simulink library "Tube_Alpha"  (R2019b)
settings: Solver=ode45  StartTime=0.0  StopTime=10.0  RelTol=1e-3  EnableMultiTasking=on
undefined symbols (not defined in the file): Tube
libraries: simulink x1
settings Model: Creator=mbrauer  LastModifiedBy=bhisma
settings DataIOCC: LimitDataPoints=on  SaveFormat=Array  SignalLoggingSaveFormat=ModelDataLogs  ReturnWorkspaceOutputs=off
settings OptimizationCC: LifeSpan=inf
settings DebuggingCC: UnderspecifiedInitializationDetection=Classic  MergeDetectMultiDrivingBlocksExec=none  SolverPrmCheckMsg=warning  MultiTaskDSMMsg=warning  MultiTaskCondExecSysMsg=none  SFUnexpectedBacktrackingDiag=warning  SFNoUnconditionalDefaultTransitionDiag=warning  SFExecutionAtInitializationDiag=none  ArithmeticOperatorsInVariantConditions=warning
settings HardwareCC: ProdBitPerPointer=32  ProdBitPerSizeT=32  ProdBitPerPtrDiffT=32  ProdLargestAtomicFloat=None  ProdIntDivRoundTo=Undefined  ProdEndianess=Unspecified  ProdWordSize=32  ProdHWDeviceType=32-bit Generic
settings ModelReferenceCC: PropagateSignalLabelsOutOfModel=off
settings SFSimCC: SimUseLocalCustomCode=off  CustomCodeUndefinedFunction=UseInterfaceOnly
settings RTWCC: RTWUseLocalCustomCode=off
settings CodeAppCC: StateflowObjectComments=on
settings GRTTargetCC: TargetLangStandard=C89/C90 (ANSI)  GeneratePreprocessorConditionals=Disable all
settings ConfigComp: CovMetricSettings=dw  CovHtmlReporting=on  CovSaveCumulativeToWorkspaceVar=on  CovSaveSingleToWorkspaceVar=on  CovExternalEMLEnable=off

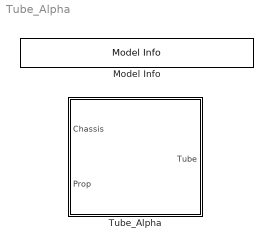
== system Tube_Alpha ==
  Model Info : simulink/Model-Wide Utilities/Model Info  Frame=on  DisplayStringWithTags=Copyright 2013-2014 The MathWorks, Inc.  HorizontalTextAlignment=Center  LeftAlignmentValue=0.5
  Tube_Alpha : Subsystem  VariantControl=VAR_Tube_Alpha

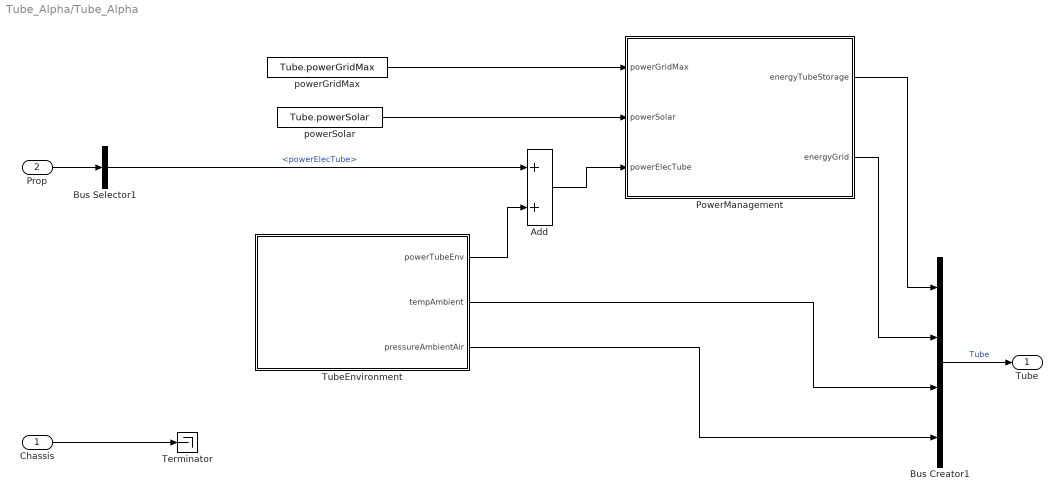
== system Tube_Alpha/Tube_Alpha ==
  Chassis : Inport
  Prop : Inport  Port=2
  Add : Sum
  Bus Creator1 : BusCreator  Inputs=4  NonVirtualBus=on
  Bus Selector1 : BusSelector  OutputSignals=powerElecTube
  PowerManagement : Subsystem
  Terminator : Terminator
  TubeEnvironment : Subsystem
  powerGridMax : Constant  Value=Tube.powerGridMax
  powerSolar : Constant  Value=Tube.powerSolar
  Tube : Outport
  wires:
  TubeEnvironment/2(tempAmbient) -> Bus Creator1/3
  Bus Creator1/1 -> Tube/1  "Tube"
  PowerManagement/1(energyTubeStorage) -> Bus Creator1/1
  Prop/1 -> Bus Selector1/1
  TubeEnvironment/1(powerTubeEnv) -> Add/2
  PowerManagement/2(energyGrid) -> Bus Creator1/2
  TubeEnvironment/3(pressureAmbientAir) -> Bus Creator1/4
  powerSolar/1 -> PowerManagement/2(powerSolar)
  powerGridMax/1 -> PowerManagement/1(powerGridMax)
  Bus Selector1/1 -> Add/1  "<powerElecTube>"
  Add/1 -> PowerManagement/3(powerElecTube)
  Chassis/1 -> Terminator/1

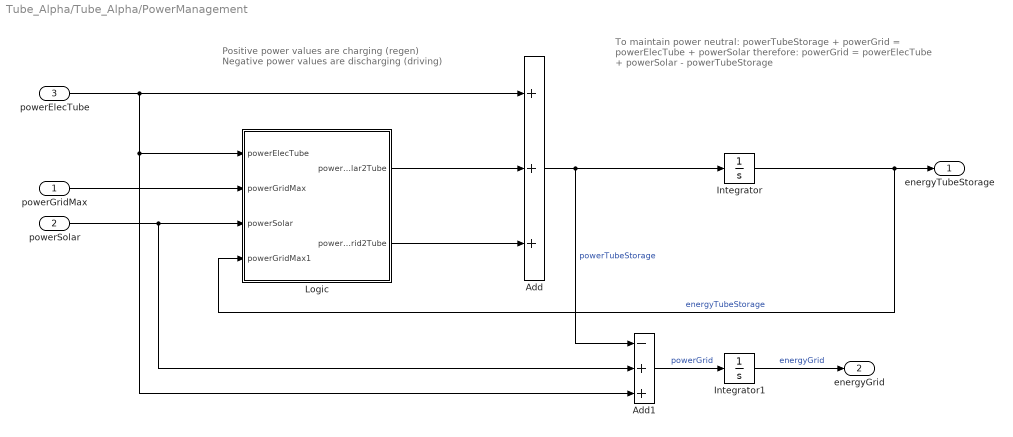
== system Tube_Alpha/Tube_Alpha/PowerManagement ==
  note: To maintain power neutral:
      | powerTubeStorage + powerGrid = powerElecTube + powerSolar
      |
      | therefore:
      | powerGrid = powerElecTube + powerSolar - powerTubeStorage
  note: Positive power values are charging (regen)
      | Negative power values are discharging (driving)
  powerGridMax : Inport
  powerSolar : Inport  Port=2
  powerElecTube : Inport  Port=3
  Add : Sum  Inputs=+++
  Add1 : Sum  Inputs=-++
  Integrator : Integrator  InitialCondition=Tube.energyStorage
      settings: AttributesFormatString=IC = %<InitialCondition>
  Integrator1 : Integrator
      settings: AttributesFormatString=IC = %<InitialCondition>
  Logic : Subsystem
  energyTubeStorage : Outport
  energyGrid : Outport  Port=2
  wires:
  Add/1 -> Integrator/1, Add1/1  "powerTubeStorage"
  Integrator1/1 -> energyGrid/1  "energyGrid"
  powerElecTube/1 -> Add1/3, Logic/1(powerElecTube), Add/1
  Integrator/1 -> Logic/4(powerGridMax1), energyTubeStorage/1  "energyTubeStorage"
  powerSolar/1 -> Add1/2, Logic/3(powerSolar)
  Add1/1 -> Integrator1/1  "powerGrid"
  powerGridMax/1 -> Logic/2(powerGridMax)
  Logic/1(powerSolar2Tube) -> Add/2
  Logic/2(powerGrid2Tube) -> Add/3

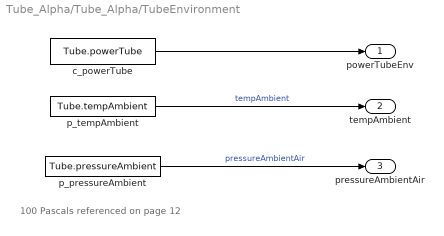
== system Tube_Alpha/Tube_Alpha/TubeEnvironment ==
  note: 100 Pascals referenced on page 12
  c_powerTube : Constant  Value=Tube.powerTube
  p_pressureAmbient : Constant  Value=Tube.pressureAmbient
  p_tempAmbient : Constant  Value=Tube.tempAmbient
  powerTubeEnv : Outport
  tempAmbient : Outport  Port=2
  pressureAmbientAir : Outport  Port=3
  wires:
  p_tempAmbient/1 -> tempAmbient/1  "tempAmbient"
  p_pressureAmbient/1 -> pressureAmbientAir/1  "pressureAmbientAir"
  c_powerTube/1 -> powerTubeEnv/1

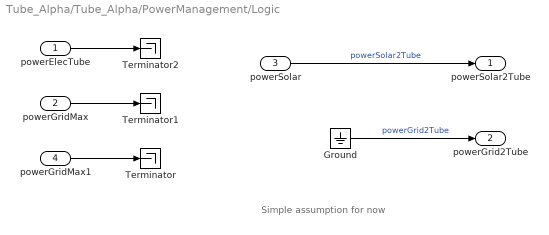
== system Tube_Alpha/Tube_Alpha/PowerManagement/Logic ==
  note: Simple assumption for now
  powerElecTube : Inport
  powerGridMax : Inport  Port=2
  powerSolar : Inport  Port=3
  powerGridMax1 : Inport  Port=4
  Ground : Ground
  Terminator : Terminator
  Terminator1 : Terminator
  Terminator2 : Terminator
  powerSolar2Tube : Outport
  powerGrid2Tube : Outport  Port=2
  wires:
  powerElecTube/1 -> Terminator2/1
  powerGridMax/1 -> Terminator1/1
  powerSolar/1 -> powerSolar2Tube/1  "powerSolar2Tube"
  Ground/1 -> powerGrid2Tube/1  "powerGrid2Tube"
  powerGridMax1/1 -> Terminator/1
